simulink model "P5_amp_rob_manipuladores"  (R2023b)
settings: Solver=VariableStepAuto  StartTime=0.0  StopTime=10  RelTol=1e-3
settings Model: Creator=Usuario_UMA  LastModifiedBy=Usuario_UMA

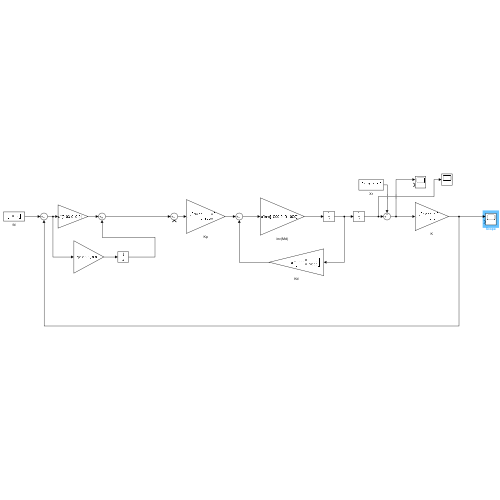
[thumbnail: Simulink's stored preview of the top-level diagram]
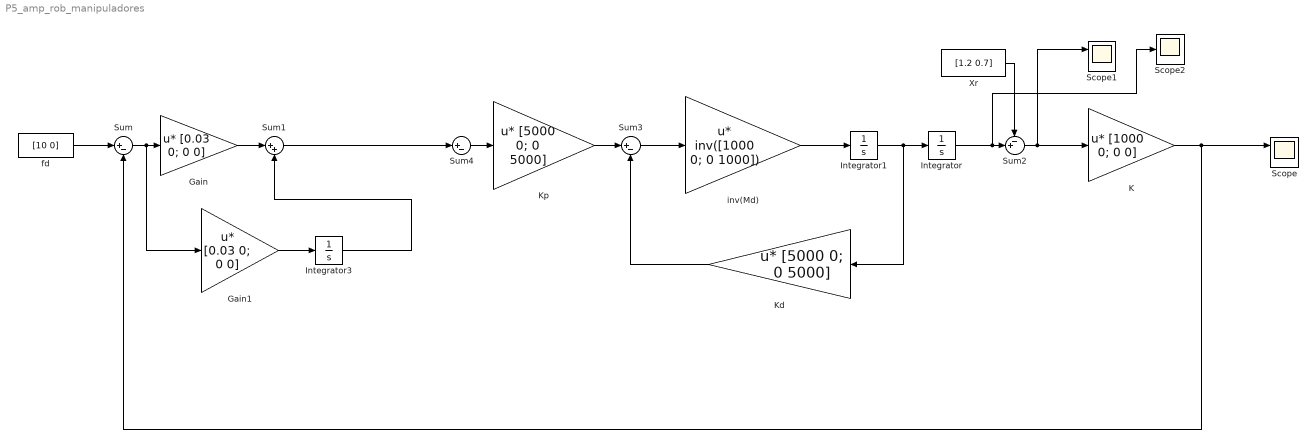
== system P5_amp_rob_manipuladores ==
  Gain : Gain  Gain=[0.03 0; 0 0]  Multiplication=Matrix(u*K)
  Gain1 : Gain  Gain=[0.03 0; 0 0]  Multiplication=Matrix(u*K)
  Integrator : Integrator  InitialCondition=[1.3 0.7]
  Integrator1 : Integrator  InitialCondition=[0 0]
  Integrator3 : Integrator
  K : Gain  Gain=[1000 0; 0 0]  Multiplication=Matrix(u*K)
  Kd : Gain  Gain=[5000 0; 0 5000]  Multiplication=Matrix(u*K)
  Kp : Gain  Gain=[5000 0; 0 5000]  Multiplication=Matrix(u*K)
  Scope : Scope  NumInputPorts=2
  Scope1 : Scope  NumInputPorts=2
  Scope2 : Scope
  Sum : Sum  Inputs=|+-
  Sum1 : Sum  Inputs=|++
  Sum2 : Sum  Inputs=-+|
  Sum3 : Sum  Inputs=|+-
  Sum4 : Sum  Inputs=|+-
  Xr : Constant  Value=[1.2 0.7]
  fd : Constant  Value=[10 0]
  inv(Md) : Gain  Gain=inv([1000 0; 0 1000])  Multiplication=Matrix(u*K)
  wires:
  fd/1 -> Sum/1
  Sum/1 -> Gain1/1, Gain/1
  Sum4/1 -> Kp/1
  Kp/1 -> Sum3/1
  Sum2/1 -> Scope1/1, K/1
  K/1 -> Scope/1, Sum/2
  Integrator/1 -> Scope2/1, Sum2/2
  Integrator1/1 -> Kd/1, Integrator/1
  Kd/1 -> Sum3/2
  inv(Md)/1 -> Integrator1/1
  Sum3/1 -> inv(Md)/1
  Xr/1 -> Sum2/1
  Gain1/1 -> Integrator3/1
  Integrator3/1 -> Sum1/2
  Gain/1 -> Sum1/1
  Sum1/1 -> Sum4/1
